simulink model "sltbu"  (Simulink 8.7)
settings: Solver=ode3  SolverMode=SingleTasking  StartTime=0.0  StopTime=999999  FixedStep=0.1  MaxStep=0.1  RelTol=1e-3  AbsTol=1e-6
PreLoadFcn:
  | inittbu;
undefined symbols (not defined in the file or in its folder): backup_speed, truck_l
undefined symbols (not defined in the file): TbuInitCond
libraries: fuzblock x1
CloseFcn:
  | [winName] = get_param(0, 'CurrentSystem'); AnimFigTitle = [winName, ': Truck Backer-Upper Animation']; AnimFigH = findobj(0,'Name',AnimFigTitle); close(AnimFigH)
settings Model: FPTRunName=Active  Creator=pascal  LastModifiedBy=FuYaqiong
settings DataIOCC: LimitDataPoints=off  SignalLoggingSaveFormat=ModelDataLogs  SaveOutput=off  SaveTime=off
settings OptimizationCC: BlockReduction=off  BooleanDataType=off  ExpressionDepthLimit=2147483647  InitFltsAndDblsToZero=on
settings DebuggingCC: SaveWithParameterizedLinksMsg=none  SignalResolutionControl=TryResolveAllWithWarning  MultiTaskDSMMsg=warning  MultiTaskCondExecSysMsg=none  FcnCallInpInsideContextMsg=UseLocalSettings  StateNameClashWarn=warning  StrictBusMsg=None
settings HardwareCC: TargetUnknown=on
settings RTWCC: TemplateMakefile=grt_vc.tmf
settings GRTTargetCC: TargetFcnLib=ansi_tfl_tmw.mat  CombineOutputUpdateFcns=off  GRTInterface=on

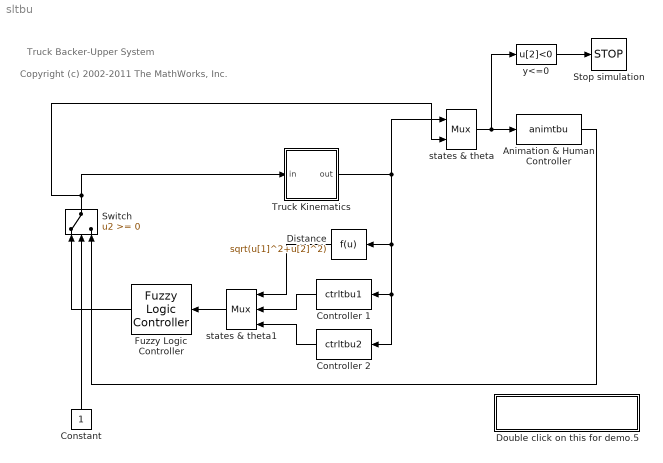
== system sltbu ==
  note: Copyright (c) 2002-2011 The MathWorks, Inc.
  note: Truck Backer-Upper System
  " Animation & Human Controller" : S-Function  FunctionName=animtbu  SFunctionDeploymentMode=off  EnableBusSupport=off
  Constant : Constant
  Controller 1 : MATLABFcn  MATLABFcn=ctrltbu1  OutputDimensions=1
  Controller 2 : MATLABFcn  MATLABFcn=ctrltbu2  OutputDimensions=1
  Distance : Fcn  Expr=sqrt(u[1]^2+u[2]^2)
  Double click on this for demo.5 : Subsystem
      settings: OpenFcn=inittbu
      mask Display: disp('Variable Initialization')
  Fuzzy Logic Controller : fuzblock/Fuzzy Logic  Controller  fis=fismat
  Stop simulation : Stop
  Switch : Switch  SaturateOnIntegerOverflow=on  InputSameDT=on
  Truck Kinematics : Subsystem  mask(Truck Dynamics){init_cond=TbuInitCond, backup_speed=backup_speed, truck_l=truck_l}
      mask prompts: init_cond "Initial Conditions (x, y, phi):"; backup_speed "Backup Speed:"; truck_l "truck Length:"
      mask help: Truck Dynamics
      mask Help: Truck dynamics
      mask Display: plot(-3, -3, 3, 3,[-1 1 1 -1 -1],[-2 -2 2 2 -2],[-1.1 -1.1],[-2 -1],[1.1 1.1],[-2 -1],[1.35 0.85],[1.93 1.07],[-0.85 -1.35],[1.93 1.07])
  states & theta : Mux  Inputs=[3 1]
  states & theta1 : Mux  Inputs=3
  y<=0 : Fcn  Expr=u[2]<0
  wires:
  y<=0/1 -> Stop simulation/1
  Switch/1 -> Truck Kinematics/1(in), states & theta/2
  Truck Kinematics/1(out) -> states & theta/1, Distance/1, Controller 1/1, Controller 2/1
  Constant/1 -> Switch/2
  states & theta/1 -> " Animation & Human Controller"/1, y<=0/1
  Fuzzy Logic Controller/1 -> Switch/1
  " Animation & Human Controller"/1 -> Switch/3
  states & theta1/1 -> Fuzzy Logic Controller/1
  Distance/1 -> states & theta1/1
  Controller 1/1 -> states & theta1/2
  Controller 2/1 -> states & theta1/3

== system sltbu/Double click on this for demo.5 ==

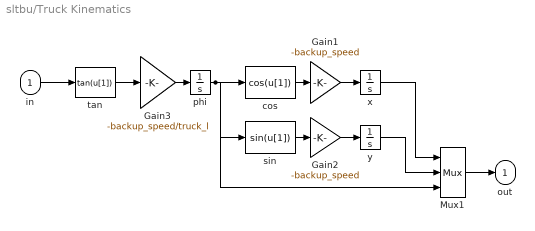
== system sltbu/Truck Kinematics ==
  in : Inport
  Gain1 : Gain  Gain=-backup_speed  SaturateOnIntegerOverflow=on  OutDataTypeStr=Inherit: Same as input  ParamDataTypeStr=Inherit: Same as input
  Gain2 : Gain  Gain=-backup_speed  SaturateOnIntegerOverflow=on  OutDataTypeStr=Inherit: Same as input  ParamDataTypeStr=Inherit: Same as input
  Gain3 : Gain  Gain=-backup_speed/truck_l  SaturateOnIntegerOverflow=on  OutDataTypeStr=Inherit: Same as input  ParamDataTypeStr=Inherit: Same as input
  Mux1 : Mux  Inputs=3
  cos : Fcn  Expr=cos(u[1])
  phi : Integrator  InitialCondition=init_cond(3)
  sin : Fcn
  tan : Fcn  Expr=tan(u[1])
  x : Integrator  InitialCondition=init_cond(1)
  y : Integrator  InitialCondition=init_cond(2)
  out : Outport  InitialOutput=0
  wires:
  in/1 -> tan/1
  phi/1 -> cos/1, sin/1, Mux1/3
  cos/1 -> Gain1/1
  Gain1/1 -> x/1
  sin/1 -> Gain2/1
  Gain2/1 -> y/1
  tan/1 -> Gain3/1
  Gain3/1 -> phi/1
  Mux1/1 -> out/1
  x/1 -> Mux1/1
  y/1 -> Mux1/2
